simulink model "PID_DELTA"  (R2018b)
settings: Solver=VariableStepAuto  StartTime=0.0  StopTime=20  FixedStep=0.001  RelTol=1e-3
model workspace (MAT data in the model file):
  I_bc = 0.466666666667
  I_bi = 2.46666666667
  I_brake = 1
  I_m = 1
  R = 0.63
  b = 2
  ee = [0; 0; -2.1944]
  k_r = 1
  l_A = 1
  l_B = 2
  m_b = 1
  m_br = 1.13333333333
  m_c = 0
  m_fb = 0.2
  m_n = 1
  m_nt = 3.6
  m_p = 0
  r_Gb = 0.558823529412
  r_l = 0.63
  r_m = 0.666666666667
  theta = [0 2.09439510239 4.18879020479]
settings Model: Creator=enrico  LastModifiedBy=enrico

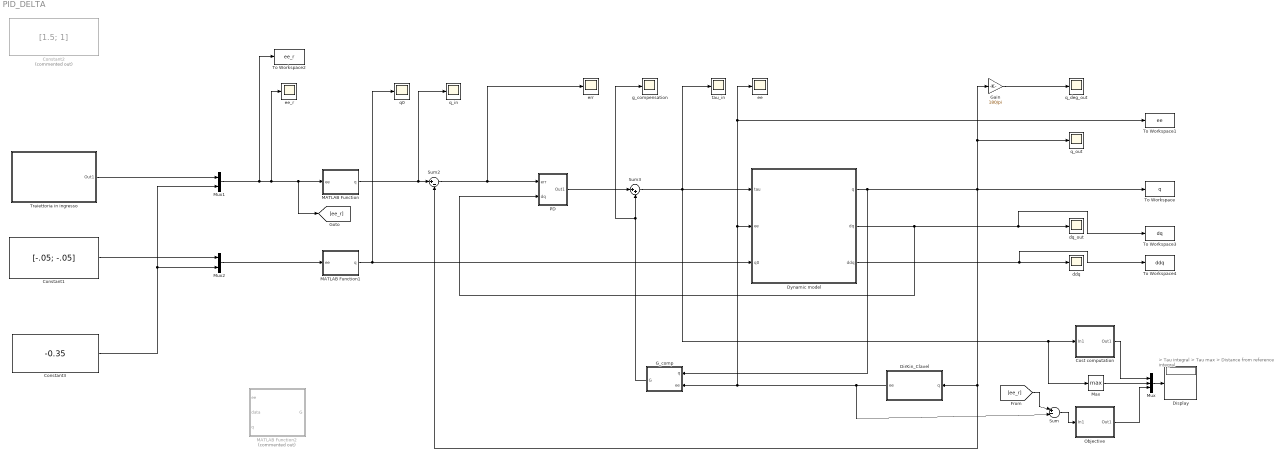
== system PID_DELTA ==
  note: > Tau integral
      |                         > Tau max
      |                         > Distance from reference
      |                            integral
  Constant1 : Constant  Value=[-.05; -.05]
  Constant2 : Constant  Commented=on  Value=[1.5; 1]
  Constant3 : Constant  Value=-0.35
  Cost computation : Subsystem
  DirKin_Clavel : MATLAB Function  TreatAsAtomicUnit=on
      mask init:
      | loadvar
  Display : Display
  Dynamic model : Subsystem
  G_comp : MATLAB Function  TreatAsAtomicUnit=on
  Gain : Gain  Gain=180/pi
  MATLAB Function : MATLAB Function  TreatAsAtomicUnit=on
  MATLAB Function1 : MATLAB Function  TreatAsAtomicUnit=on
  MATLAB Function2 : MATLAB Function  Commented=on  TreatAsAtomicUnit=on
  Max : MinMax  Function=max
  Mux : Mux  Inputs=3
  Mux1 : Mux  Inputs=2
  Mux2 : Mux  Inputs=2
  Objective : Subsystem
  PD : Subsystem  mask{Kpx=1500, Kpy=1500, Kpz=1500, D=60}
      mask prompts: D "Derivative_gain"
  Sum : Sum  Inputs=|+-|
  Sum2 : Sum  Inputs=|+-
  Sum3 : Sum  Inputs=|++
  To Workspace : ToWorkspace  VariableName=q  SampleTime=-1
  To Workspace1 : ToWorkspace  VariableName=ee  SampleTime=-1
  To Workspace2 : ToWorkspace  VariableName=ee_r  SampleTime=-1
  To Workspace3 : ToWorkspace  VariableName=dq  SampleTime=-1
  To Workspace4 : ToWorkspace  VariableName=ddq  SampleTime=-1
  Traiettoria in ingresso : Subsystem  mask{F=3, A=.05}
      mask prompts: F "Frequenza"; A "Ampiezza"
  ddq : Scope
  "dq_out " : Scope
  "ee " : Scope
  ee_r : Scope
  err : Scope
  "g_compensation " : Scope
  "q0 " : Scope
  "q_deg_out " : Scope
  q_in : Scope
  q_out : Scope
  tau_in : Scope
  wires:
  Dynamic model/2(dq) -> PD/2(dq), To Workspace3/1, "dq_out "/1
  DirKin_Clavel/1(ee) -> Sum/2, To Workspace1/1, "ee "/1, Dynamic model/2(ee), G_comp/2(ee)
  Gain/1 -> "q_deg_out "/1
  Dynamic model/3(ddq) -> To Workspace4/1, ddq/1
  Constant1/1 -> Mux2/1
  Dynamic model/1(q) -> G_comp/1(q), q_out/1, Gain/1, To Workspace/1, Sum2/2, DirKin_Clavel/1(q)
  MATLAB Function/1(q) -> Sum2/1, q_in/1
  MATLAB Function1/1(q) -> Dynamic model/3("q0 "), "q0 "/1
  G_comp/1(G) -> Sum3/2, "g_compensation "/1
  PD/1(Out1) -> Sum3/1
  Sum2/1 -> err/1, PD/1(err)
  Mux2/1 -> MATLAB Function1/1(ee)
  Constant3/1 -> Mux1/2, Mux2/2
  Traiettoria in ingresso/1(Out1) -> Mux1/1
  Sum3/1 -> Dynamic model/1(tau), Max/1, Cost computation/1(In1), tau_in/1
  Cost computation/1(Out1) -> Mux/1
  Mux1/1 -> To Workspace2/1, ee_r/1, [ee_r], MATLAB Function/1(ee)
  Sum/1 -> Objective/1(In1)
  [ee_r] -> Sum/1
  Objective/1(Out1) -> Mux/3
  Mux/1 -> Display/1
  Max/1 -> Mux/2

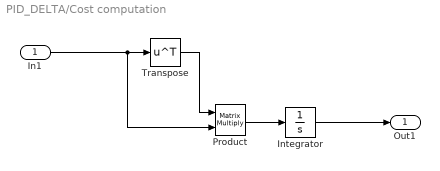
== system PID_DELTA/Cost computation ==
  In1 : Inport
  Integrator : Integrator
  Product : Product  Multiplication=Matrix(*)
  Transpose : Math  Operator=transpose  SaturateOnIntegerOverflow=on
  Out1 : Outport
  wires:
  Transpose/1 -> Product/1
  Integrator/1 -> Out1/1
  Product/1 -> Integrator/1
  In1/1 -> Product/2, Transpose/1

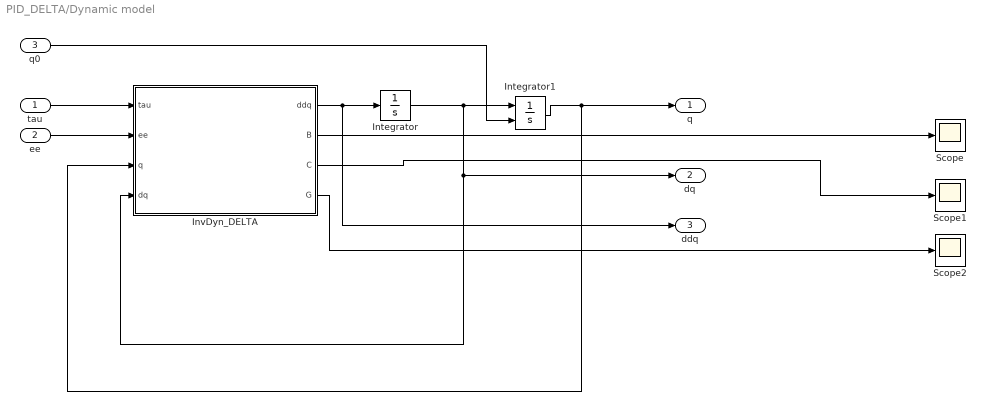
== system PID_DELTA/Dynamic model ==
  tau : Inport
  ee : Inport  Port=2
  "q0 " : Inport  Port=3
  Integrator : Integrator  InitialCondition=[0; 0; 0]
  Integrator1 : Integrator  InitialConditionSource=external  InitialCondition=[pi/4; pi/4; pi/4]
  InvDyn_DELTA : MATLAB Function  TreatAsAtomicUnit=on
  Scope : Scope
  Scope1 : Scope
  Scope2 : Scope
  q : Outport
  dq : Outport  Port=2
  ddq : Outport  Port=3
  wires:
  InvDyn_DELTA/1(ddq) -> ddq/1, Integrator/1
  ee/1 -> InvDyn_DELTA/2(ee)
  Integrator1/1 -> q/1, InvDyn_DELTA/3(q)
  Integrator/1 -> Integrator1/1, dq/1, InvDyn_DELTA/4(dq)
  tau/1 -> InvDyn_DELTA/1(tau)
  "q0 "/1 -> Integrator1/2
  InvDyn_DELTA/2(B) -> Scope/1
  InvDyn_DELTA/3(C) -> Scope1/1
  InvDyn_DELTA/4(G) -> Scope2/1

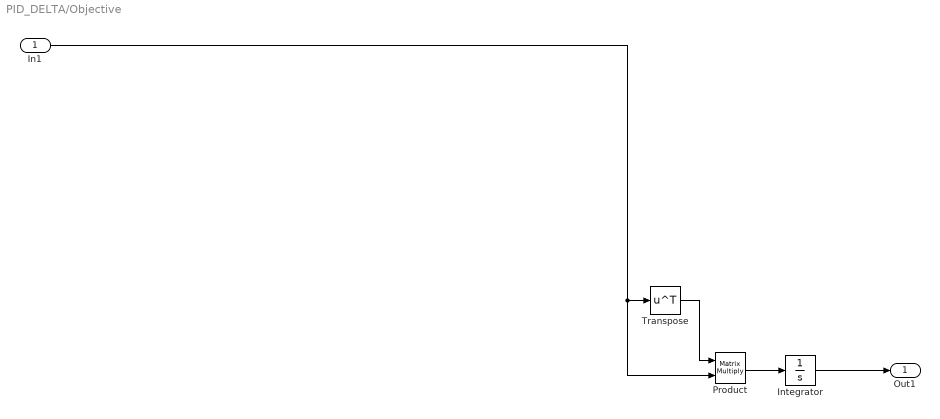
== system PID_DELTA/Objective ==
  In1 : Inport
  Integrator : Integrator
  Product : Product  Multiplication=Matrix(*)
  Transpose : Math  Operator=transpose  SaturateOnIntegerOverflow=on
  Out1 : Outport
  wires:
  In1/1 -> Transpose/1, Product/2
  Product/1 -> Integrator/1
  Integrator/1 -> Out1/1
  Transpose/1 -> Product/1

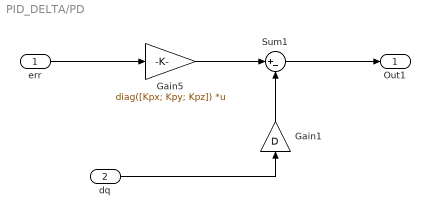
== system PID_DELTA/PD ==
  err : Inport
  dq : Inport  Port=2
  Gain1 : Gain  Gain=D
  Gain5 : Gain  Gain=diag([Kpx; Kpy; Kpz])  Multiplication=Matrix(K*u) (u vector)
  Sum1 : Sum  Inputs=|+-
  Out1 : Outport
  wires:
  Gain1/1 -> Sum1/2
  Sum1/1 -> Out1/1
  dq/1 -> Gain1/1
  err/1 -> Gain5/1
  Gain5/1 -> Sum1/1

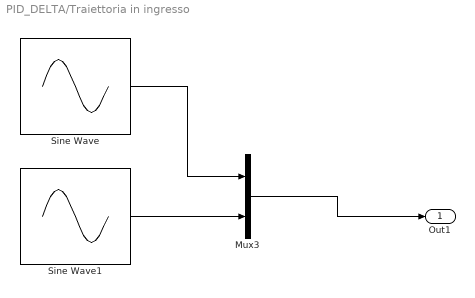
== system PID_DELTA/Traiettoria in ingresso ==
  Mux3 : Mux  Inputs=2
  Sine Wave : Sin  Amplitude=A  Frequency=F  Phase=pi/2  SampleTime=0
  Sine Wave1 : Sin  Amplitude=A  Frequency=F  SampleTime=0
  Out1 : Outport
  wires:
  Sine Wave/1 -> Mux3/1
  Sine Wave1/1 -> Mux3/2
  Mux3/1 -> Out1/1

== matlab function PID_DELTA/MATLAB Function1 ==
  data: ee input; q output
function q = InverseKinematic(ee)
%Computation of the inverse kinematic of the Delta robot

% Loading parameters
[theta, R, ~, ~, l_A, ~, ~, l_B, ~, ~, ~] = Parameters_DELTA;

R_b1 = R_base(theta(1));
R_b2 = R_base(theta(2));
R_b3 = R_base(theta(3));
p = [R_b1\ee, R_b2\ee, R_b3\ee]; 
q = nan(3,1);

for li=1:3
    
    x0 = p(1,li);
    y0 = p(2,li);
    z0 = p(3,li);
    A = l_A^2 - l_B^2 - R^2 + x0^2 + y0^2 + z0^2;
    B = 2*x0 - 2*R;

    a = 4*z0^2 + B^2;
    b = 4*R*z0^2 + A*B;
    c = A^2 + 4*R^2*z0^2 - 4*l_A^2*z0^2;
        
    x = (b + sqrt(b^2 - a*c))/a; 
    
    z = (A - B*x)/(2*z0);
    
    q(li) = - asin(z/l_A); 
    
    if x-R < 0
        q(li) = pi - q(li);
    end    
end

end

== matlab function PID_DELTA/Dynamic model/InvDyn_DELTA ==
  data: tau input; ddq output; ee input; q input; dq input; B output; C output; G output
function [ddq, B, C, G] = InvDyn_DELTA(tau, ee, q, dq)
% References:
% [1] Olsson, A. (2009). Modelling and control of a Delta-3 robot, (February).
% [2] Codourey, A. (1998). Dynamic Modeling of Parallel Robots for Computed-Torque Control Implementation, 17(12), 1325–1336.

% B, C, G matrices
[B, C, G] = BCG_DELTA(ee,q);
F = 0.7;

% Inverse dynamic
ddq = B\(tau - C*dq - G - F*dq); % Think adding friction coefficient of the manipulator (from [1] pg 27) 


end

== matlab function PID_DELTA/DirKin_Clavel ==
  data: q input; ee output
function ee = DirKin_Clavel(q)

[theta, R, ~, ~, l_A, ~, ~, l_B, ~, ~, ~] = Parameters_DELTA;

D = nan(3,1);
E = nan(3,1);
F = nan(3,1);
G = nan(3,1);

for i = 1:3
   D(i) = -l_B^2 + l_A^2 + R^2 + 2*R*l_A*cos(q(i));
   
   E(i) = 2*(R + l_A*cos(q(i)))*cos(theta(i));
   
   F(i) = 2*(R + l_A*cos(q(i)))*sin(theta(i));
   
   G(i) = -2*l_A*sin(q(i)); 
end

H = [E(1)*G(2) - E(1)*G(3) - E(2)*G(1) + E(2)*G(3) + E(3)*G(1) - E(3)*G(2);
    -E(1)*F(2) + E(1)*F(3) + E(2)*F(1) - E(2)*F(3) - E(3)*F(1) + E(3)*F(2);
    -E(1)*D(2) + E(1)*D(3) + E(2)*D(1) - E(2)*D(3) - E(3)*D(1) + E(3)*D(2);
     F(1)*D(2) - F(1)*D(3) - F(2)*D(1) + F(2)*D(3) + F(3)*D(1) - F(3)*D(2);
    -F(1)*G(2) + F(1)*G(3) + F(2)*G(1) - F(2)*G(3) - F(3)*G(1) + F(3)*G(2)];

L = (H(5)^2 + H(1)^2)/H(2)^2 + 1;

M = 2*(H(5)*H(4) + H(1)*H(3))/H(2)^2 - (H(5)*E(1) + H(1)*F(1))/H(2) - G(1);

N = (H(4)^2 + H(3)^2)/H(2)^2 - (H(4)*E(1) + H(3)*F(1))/H(2) + D(1);

ee = nan(3,1);
ee2 = nan(3,1);

ee(3) = (-M + sqrt(M^2 - 4*L*N))/(2*L);

ee(1) = ee(3)*H(5)/H(2) + H(4)/H(2);

ee(2) = ee(3)*H(1)/H(2) + H(3)/H(2);

ee2(3) = (-M - sqrt(M^2 - 4*L*N))/(2*L);

ee2(1) = ee2(3)*H(5)/H(2) + H(4)/H(2);

ee2(2) = ee2(3)*H(1)/H(2) + H(3)/H(2);
 


% if ee2(3) < 0 
%     ee = ee2;
% end

if ee(3) > ee2(3)
    ee = ee2;
end

end

== matlab function PID_DELTA/MATLAB Function ==
  data: ee input; q output
function q = InverseKinematic(ee)
%Computation of the inverse kinematic of the Delta robot

% Loading parameters
[theta, R, ~, ~, l_A, ~, ~, l_B, ~, ~, ~] = Parameters_DELTA;

R_b1 = R_base(theta(1));
R_b2 = R_base(theta(2));
R_b3 = R_base(theta(3));
p = [R_b1\ee, R_b2\ee, R_b3\ee]; 
q = nan(3,1);

for li=1:3
    
    x0 = p(1,li);
    y0 = p(2,li);
    z0 = p(3,li);
    A = l_A^2 - l_B^2 - R^2 + x0^2 + y0^2 + z0^2;
    B = 2*x0 - 2*R;

    a = 4*z0^2 + B^2;
    b = 4*R*z0^2 + A*B;
    c = A^2 + 4*R^2*z0^2 - 4*l_A^2*z0^2;
        
    x = (b + sqrt(b^2 - a*c))/a; 
    
    z = (A - B*x)/(2*z0);
    
    q(li) = - asin(z/l_A); 
    
    if x-R < 0
        q(li) = pi - q(li);
    end    
end

end

== matlab function PID_DELTA/MATLAB Function2 ==
  data: ee input; data input; G output; q input
function G = G_DELTA(ee, data, q)
%UNTITLED6 Summary of this function goes here
%   Detailed explanation goes here

[theta, ~, ~, m_br, ~, r_Gb, ~, ~, ~, m_nt, I_bi] = Parameters_DELTA;

% Arms intertia matrix
I_b = diag([I_bi, I_bi, I_bi]);

% Jacobian and its derivative
[J, dJ] = Jacobian_DELTA(ee,q);

% Inertia elements matrix
B = (I_b + m_nt*(J'*J)); 

% Coriolis elements matrix
C = (J'*m_nt*dJ);

% Gravitational elements matrix
G_n = m_nt*[0; 0; -9.81];
G_b = m_br*[0; 0; -9.81];

% tau_b =  r_Gb*[ cos(theta(1)); cos(theta(2)); -m_br*9.8*cos(theta(3))];

tau_Gb =  r_Gb*9.81*m_br*[ cos(q(1)); cos(q(2)); cos(q(3))];

G = (J'*G_n + tau_Gb);

end

== matlab function PID_DELTA/G_comp ==
  data: q input; G output; ee input
function G = fcn(q,ee)

[~, ~, ~, m_br, ~, r_Gb, ~, ~, ~, m_nt, ~] = Parameters_DELTA;

% Jacobian and its derivative
[J, ~] = Jacobian_DELTA(ee,q);

% Gravitational elements matrix
G_n = m_nt*[0; 0; -9.81];
% G_b = m_br*[0; 0; -9.81];

% tau_b =  r_Gb*[ cos(theta(1)); cos(theta(2)); -m_br*9.8*cos(theta(3))];

tau_Gb =  r_Gb*9.81*m_br*[ cos(q(1)); cos(q(2)); cos(q(3))];

G = (J'*G_n + tau_Gb);

end
